simulink model "hr_sunlight"  (R2017a)
settings: Solver=FixedStepAuto  StartTime=1  StopTime=1  FixedStep=1  RelTol=1e-3
libraries: simulink_extras x4
settings Model: Creator=zhiangz  LastModifiedBy=zhiangz

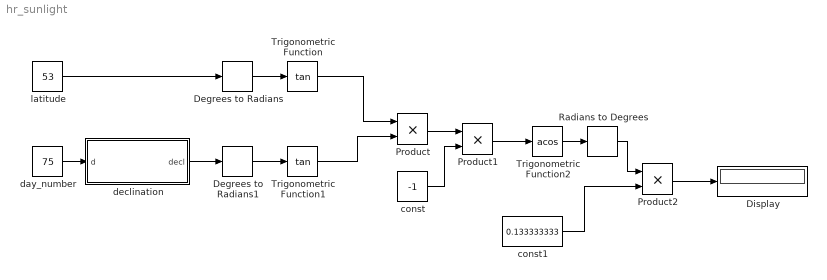
== system hr_sunlight ==
  Degrees to Radians : simulink_extras/Transformations/Degrees to Radians
  Degrees to Radians1 : simulink_extras/Transformations/Degrees to Radians
  Display : Display
      settings: Decimation=2
  Product : Product
  Product1 : Product
  Product2 : Product
  Radians to Degrees : simulink_extras/Transformations/Radians to Degrees
  Trigonometric Function : Trigonometry  Operator=tan
  Trigonometric Function1 : Trigonometry  Operator=tan
  Trigonometric Function2 : Trigonometry  Operator=acos  OutputSignalType=real
  const : Constant  Value=-1
  const1 : Constant  Value=0.133333333
  day_number : Constant  Value=75
  declination : Subsystem
  latitude : Constant  Value=53
  wires:
  day_number/1 -> declination/1(d)
  Trigonometric Function/1 -> Product/1
  Trigonometric Function1/1 -> Product/2
  Product/1 -> Product1/1
  const/1 -> Product1/2
  Product1/1 -> Trigonometric Function2/1
  const1/1 -> Product2/2
  Product2/1 -> Display/1
  Trigonometric Function2/1 -> Radians to Degrees/1
  Radians to Degrees/1 -> Product2/1
  declination/1(decl) -> Degrees to Radians1/1
  latitude/1 -> Degrees to Radians/1
  Degrees to Radians/1 -> Trigonometric Function/1
  Degrees to Radians1/1 -> Trigonometric Function1/1

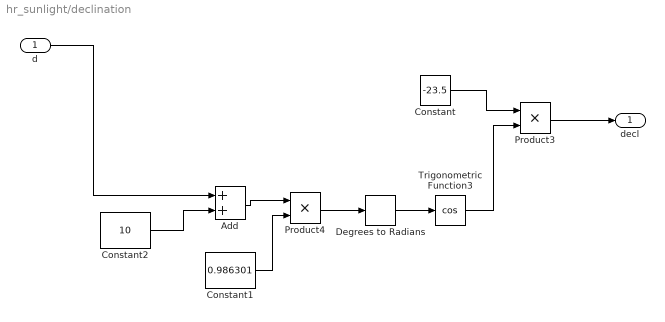
== system hr_sunlight/declination ==
  d : Inport
  Add : Sum
  Constant : Constant  Value=-23.5
  Constant1 : Constant  Value=0.986301
  Constant2 : Constant  Value=10
  Degrees to Radians : simulink_extras/Transformations/Degrees to Radians
  Product3 : Product
  Product4 : Product
  Trigonometric Function3 : Trigonometry  Operator=cos
  decl : Outport
  wires:
  Trigonometric Function3/1 -> Product3/2
  Constant1/1 -> Product4/2
  Constant/1 -> Product3/1
  Product4/1 -> Degrees to Radians/1
  Add/1 -> Product4/1
  d/1 -> Add/1
  Constant2/1 -> Add/2
  Product3/1 -> decl/1
  Degrees to Radians/1 -> Trigonometric Function3/1
